simulink model "pos2lonlat"  (R2017b)
settings: Solver=VariableStepAuto  StartTime=0.0  StopTime=10.0  RelTol=1e-3
undefined symbols (not defined in the file or in its folder): Visual
settings Model: Creator=One  LastModifiedBy=One

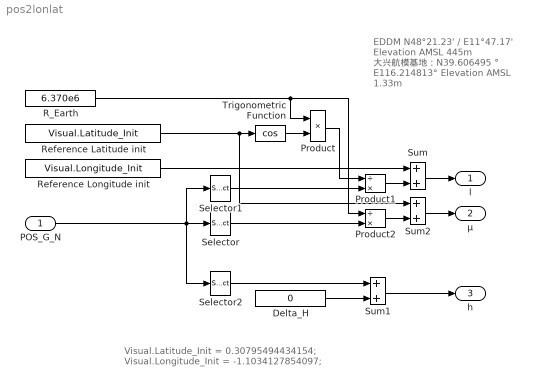
== system pos2lonlat ==
  note: EDDM N48°21.23' / E11°47.17'
      | Elevation AMSL 445m
      |
      | 大兴航模基地：N39.606495 °
      | E116.214813°
      | Elevation AMSL 1.33m
  note: Visual.Latitude_Init  = 0.30795494434154;
      | Visual.Longitude_Init = -1.1034127854097;
  POS_G_N : Inport
  Delta_H : Constant  Value=0
  Product : Product
  Product1 : Product  Inputs=/*
  Product2 : Product  Inputs=/*
  R_Earth : Constant  Value=6.370e6
  Reference Latitude init : Constant  Value=Visual.Latitude_Init
  Reference Longitude init : Constant  Value=Visual.Longitude_Init
  Selector : Selector  InputPortWidth=3  IndexOptions=Index vector (dialog)  Indices=[1]  OutputSizes=1
  Selector1 : Selector  InputPortWidth=3  IndexOptions=Index vector (dialog)  Indices=[2]  OutputSizes=1
  Selector2 : Selector  InputPortWidth=3  IndexOptions=Index vector (dialog)  Indices=[3]  OutputSizes=1
  Sum : Sum
  Sum1 : Sum
  Sum2 : Sum
  Trigonometric Function : Trigonometry  Operator=cos
  l : Outport  PortDimensions=1
  μ : Outport  Port=2  PortDimensions=1
  h : Outport  Port=3  Unit=m  PortDimensions=1
  wires:
  R_Earth/1 -> Product2/1, Product/1
  Reference Longitude init/1 -> Sum/1
  Sum2/1 -> μ/1
  Delta_H/1 -> Sum1/2
  Product2/1 -> Sum2/2
  Sum/1 -> l/1
  Product1/1 -> Sum/2
  Sum1/1 -> h/1
  Reference Latitude init/1 -> Trigonometric Function/1, Sum2/1
  Selector1/1 -> Product1/2
  Product/1 -> Product1/1
  Selector2/1 -> Sum1/1
  Selector/1 -> Product2/2
  Trigonometric Function/1 -> Product/2
  POS_G_N/1 -> Selector2/1, Selector1/1, Selector/1
